simulink model "Simulink_model_problem_5_3"  (R2023b)
settings: Solver=ode45  StartTime=0.0  StopTime=20  RelTol=1e-1
values from neighbouring files (symbols this model uses):
  shapeit_data =     [problem_5_3_controller_plant.mat]
libraries: simulink x3
settings Model: Creator=sarth  LastModifiedBy=sarth

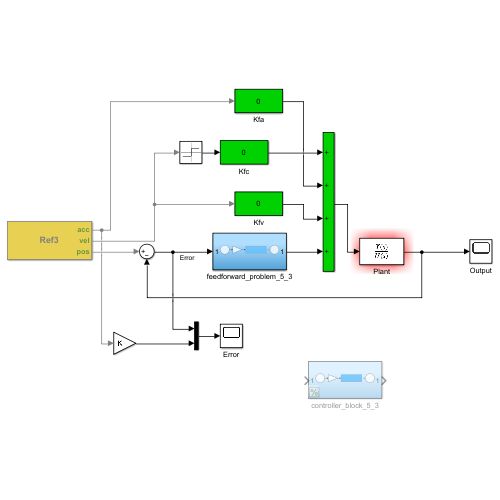
[thumbnail: Simulink's stored preview of the top-level diagram]
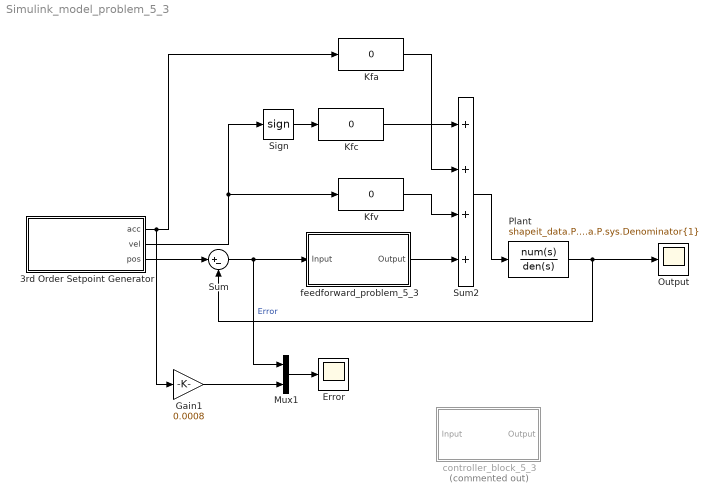
== system Simulink_model_problem_5_3 ==
  3rd Order Setpoint Generator : Subsystem  mask(Ref3){}
      settings: OpenFcn=r3g_main
      mask Display: disp('Ref3');
  Error : Scope
  Gain1 : Gain  Gain=0.0008  SaturateOnIntegerOverflow=on  OutDataTypeStr=Inherit: Same as input  ParamDataTypeStr=Inherit: Same as input
  Kfa : simulink/Math Operations/Slider Gain  gain=0  low=0  high=1
  Kfc : simulink/Math Operations/Slider Gain  gain=0  low=0  high=1
  Kfv : simulink/Math Operations/Slider Gain  gain=0  low=0  high=1
  Mux1 : Mux  Inputs=2
  Output : Scope
  Plant : TransferFcn  Numerator=shapeit_data.P.sys.Numerator{1}  Denominator=shapeit_data.P.sys.Denominator{1}
  Sign : Signum
  Sum : Sum  Inputs=|+-
  Sum2 : Sum  Inputs=++++  SaturateOnIntegerOverflow=on
  controller_block_5_3 : Subsystem  Commented=on
  feedforward_problem_5_3 : Subsystem
  wires:
  Plant/1 -> Output/1, Sum/2
  feedforward_problem_5_3/1(Output) -> Sum2/4
  Sum2/1 -> Plant/1
  3rd Order Setpoint Generator/3(pos) -> Sum/1
  Sign/1 -> Kfc/1
  Kfv/1 -> Sum2/3
  Kfa/1 -> Sum2/2
  3rd Order Setpoint Generator/2(vel) -> Kfv/1, Sign/1
  3rd Order Setpoint Generator/1(acc) -> Gain1/1, Kfa/1
  Sum/1 -> feedforward_problem_5_3/1(Input), Mux1/1  "Error"
  Mux1/1 -> Error/1
  Gain1/1 -> Mux1/2
  Kfc/1 -> Sum2/1

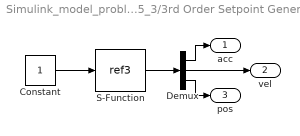
== system Simulink_model_problem_5_3/3rd Order Setpoint Generator ==
  Constant : Constant
  Demux : Demux  Outputs=3
      settings: DisplayOption=none
  S-Function : S-Function  FunctionName=ref3  Parameters=ref_part  SFunctionDeploymentMode=off  EnableBusSupport=off
      settings: OpenFcn=global ref_part; r3g_main
  acc : Outport
  vel : Outport  Port=2
  pos : Outport  Port=3
  wires:
  Constant/1 -> S-Function/1
  S-Function/1 -> Demux/1
  Demux/1 -> acc/1
  Demux/2 -> vel/1
  Demux/3 -> pos/1

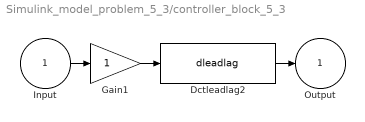
== system Simulink_model_problem_5_3/controller_block_5_3 ==
  Input : Inport
  Dctleadlag2 : S-Function  FunctionName=dleadlag  Parameters=f_num, f_den, 0.001  SFunctionDeploymentMode=off  EnableBusSupport=off  mask(dctools){f_num=1.7, f_den=15.3}
      mask prompts: f_num "Zero [Hz]"; f_den "Pole [Hz]"
      mask help: This block implements a discrete time leadlag filter.
      mask Display: disp('DCT leadlag')
  Gain1 : Gain
  Output : Outport
  wires:
  Input/1 -> Gain1/1
  Gain1/1 -> Dctleadlag2/1
  Dctleadlag2/1 -> Output/1

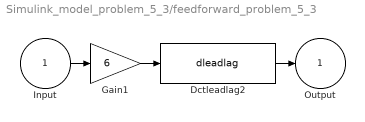
== system Simulink_model_problem_5_3/feedforward_problem_5_3 ==
  Input : Inport
  Dctleadlag2 : S-Function  FunctionName=dleadlag  Parameters=f_num, f_den, 0.001  SFunctionDeploymentMode=off  EnableBusSupport=off  mask(dctools){f_num=2.336, f_den=58.4}
      mask prompts: f_num "Zero [Hz]"; f_den "Pole [Hz]"
      mask help: This block implements a discrete time leadlag filter.
      mask Display: disp('DCT leadlag')
  Gain1 : Gain  Gain=6
  Output : Outport
  wires:
  Input/1 -> Gain1/1
  Gain1/1 -> Dctleadlag2/1
  Dctleadlag2/1 -> Output/1
